simulink model "MPC_Observer_revised2"  (R2015a)
settings: Solver=ode5  StartTime=0.0  StopTime=Total_t_sim  FixedStep=dt  RelTol=1e-3
values from neighbouring files (symbols this model uses):
  A = F    [DMPC_AVC12.m]    (also in DMPC_AVC2.m; DMPC_AVC4.m; DMPC_AVC6.m)
  A_cons = [L_m;-L_m]    [DMPC_AVC12.m]    (also in DMPC_AVC2.m; DMPC_AVC4.m; DMPC_AVC6.m)
  A_nom = A    [DMPC_AVC12.m]    (also in DMPC_AVC2.m; DMPC_AVC4.m; DMPC_AVC6.m)
  B = G    [DMPC_AVC12.m]    (also in DMPC_AVC2.m; DMPC_AVC4.m; DMPC_AVC6.m)
  B_nom = B    [DMPC_AVC12.m]    (also in DMPC_AVC2.m; DMPC_AVC4.m; DMPC_AVC6.m)
  C = H    [DMPC_AVC12.m]    (also in DMPC_AVC2.m; DMPC_AVC4.m; DMPC_AVC6.m)
  C_nom = C    [DMPC_AVC12.m]    (also in DMPC_AVC2.m; DMPC_AVC4.m; DMPC_AVC6.m)
  coefs = coefs(1,2:end)    [DMPC_AVC12.m]    (also in DMPC_AVC2.m; DMPC_AVC4.m; DMPC_AVC6.m)
  dt = 5e-4    (= 0.0005)    [DMPC_AVC12.m]    (also in DMPC_AVC2.m = 0.001; DMPC_AVC4.m = 0.001; DMPC_AVC6.m = 0.001)
  H_nom = H    [DMPC_AVC12.m]    (also in DMPC_AVC2.m; DMPC_AVC4.m; DMPC_AVC6.m)
  Lf = Kalman_Gain(A,C,Qf,Rf,Pf,Nsim,nout)    [DMPC_AVC12.m]    (also in DMPC_AVC2.m; DMPC_AVC4.m; DMPC_AVC6.m)
  u_bound = [u_max;-u_min]    [DMPC_AVC12.m]    (also in DMPC_AVC2.m; DMPC_AVC4.m; DMPC_AVC6.m)
  V = gt_modal.C    [identification_SPM_IMP.m]    (also in identified_shaker.mat = [-0.780917041134 1.13362828061])
  W = gt_modal.A    [identification_SPM_IMP.m]    (also in identified_shaker.mat = [-1.30981674822  104.165252735; -104.165252735  -1.309816748)
undefined symbols (not defined in the file or in its folder): L_m, omega, psi
libraries: simulink_need_slupdate x2
settings Model: Creator=Ablah  LastModifiedBy=Ablah

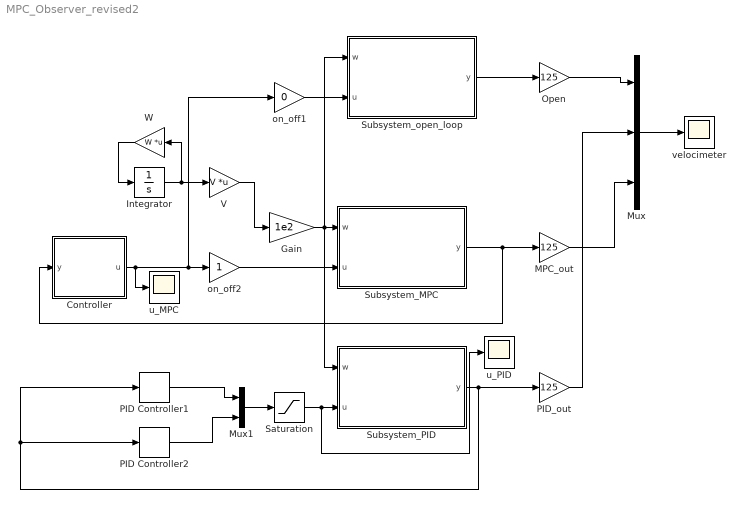
== system MPC_Observer_revised2 ==
  Controller : Subsystem
  Gain : Gain  Gain=1e2
  Integrator : Integrator  InitialCondition=0.01
  MPC_out : Gain  Gain=125
  Mux : Mux  Inputs=3
  Mux1 : Mux  Inputs=2
  Open : Gain  Gain=125
  PID Controller1 : simulink_need_slupdate/PID Controller  P=-3  I=-4  D=0
  PID Controller2 : simulink_need_slupdate/PID Controller  P=-3  I=-4  D=0
  PID_out : Gain  Gain=125
  Saturation : Saturate  UpperLimit=0.6  LowerLimit=-0.6
  Subsystem_MPC : Subsystem
  Subsystem_PID : Subsystem
  Subsystem_open_loop : Subsystem
  V : Gain  Gain=V  Multiplication=Matrix(K*u)
  W : Gain  Gain=W  Multiplication=Matrix(K*u)
  on_off1 : Gain  Gain=0
  on_off2 : Gain
  u_MPC : Scope
      settings: YMin=-2.25  YMax=2.25  SaveName=ScopeData5
  u_PID : Scope
      settings: YMin=-2.25  YMax=2.25  SaveName=ScopeData4
  velocimeter : Scope
      settings: ShowLegends=on  YMin=-10  YMax=10
  wires:
  Controller/1(u) -> u_MPC/1, on_off1/1, on_off2/1
  Gain/1 -> Subsystem_PID/1(w), Subsystem_open_loop/1(w), Subsystem_MPC/1(w)
  Subsystem_MPC/1(y) -> Controller/1(y), MPC_out/1
  on_off2/1 -> Subsystem_MPC/2(u)
  W/1 -> Integrator/1
  Integrator/1 -> V/1, W/1
  V/1 -> Gain/1
  on_off1/1 -> Subsystem_open_loop/2(u)
  Subsystem_open_loop/1(y) -> Open/1
  Mux/1 -> velocimeter/1
  Subsystem_PID/1(y) -> PID Controller2/1, PID Controller1/1, PID_out/1
  PID Controller1/1 -> Mux1/1
  Mux1/1 -> Saturation/1
  Saturation/1 -> u_PID/1, Subsystem_PID/2(u)
  PID Controller2/1 -> Mux1/2
  MPC_out/1 -> Mux/3
  Open/1 -> Mux/1
  PID_out/1 -> Mux/2

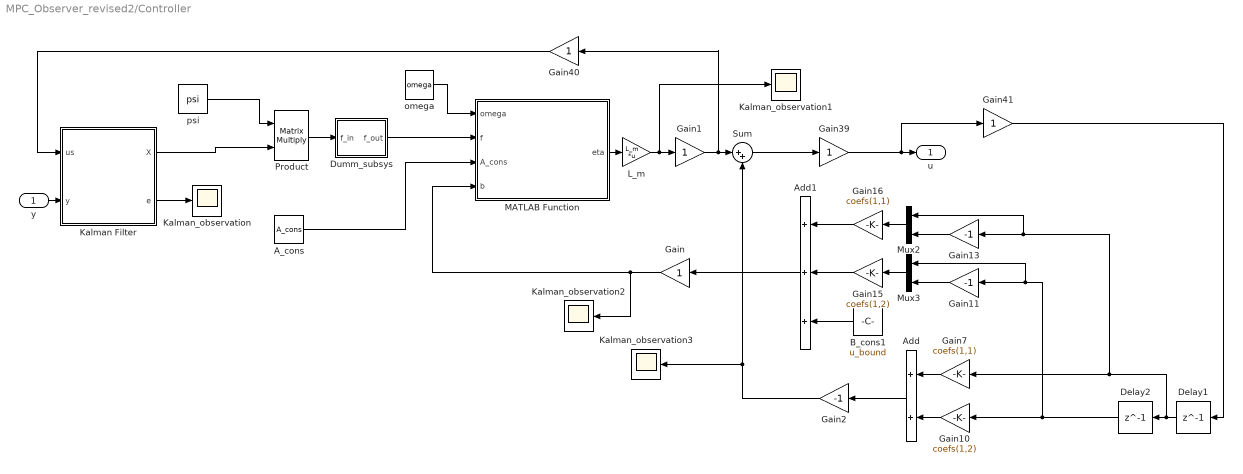
== system MPC_Observer_revised2/Controller ==
  y : Inport
  A_cons : Constant  Value=A_cons  SampleTime=dt
  Add : Sum
  Add1 : Sum  Inputs=+++
  B_cons1 : Constant  Value=u_bound
  Delay1 : Delay  DelayLength=1  InitialCondition=0  SampleTime=dt
  Delay2 : Delay  DelayLength=1  InitialCondition=0  SampleTime=dt
  Dumm_subsys : Subsystem
  Gain{,1,39..41} (5 alike) : Gain
  Gain10 : Gain  Gain=coefs(1,2)
  Gain11 : Gain  Gain=-1
  Gain13 : Gain  Gain=-1
  Gain15 : Gain  Gain=coefs(1,2)
  Gain16 : Gain  Gain=coefs(1,1)
  Gain2 : Gain  Gain=-1
  Gain7 : Gain  Gain=coefs(1,1)
  Kalman Filter : Subsystem  TreatAsAtomicUnit=on
      settings: MinAlgLoopOccurrences=on
  Kalman_observation{,1..3} (4 alike) : Scope
      Kalman_observation settings: YMin=-3.5e-11  YMax=3.5e-11
      Kalman_observation1 settings: YMin=-0.000155  YMax=-6.5e-05  SaveName=ScopeData2
      Kalman_observation2 settings: YMin=-0.000155  YMax=-6.5e-05  SaveName=ScopeData6
      Kalman_observation3 settings: YMin=-0.000155  YMax=-6.5e-05  SaveName=ScopeData7
  L_m : Gain  Gain=L_m  Multiplication=Matrix(K*u)
  MATLAB Function : MATLAB Function  TreatAsAtomicUnit=on
      settings: MinAlgLoopOccurrences=on
  Mux2 : Mux  Inputs=2
  Mux3 : Mux  Inputs=2
  Product : Product  Multiplication=Matrix(*)  RndMeth=Zero
  Sum : Sum  Inputs=|++
  omega : Constant  Value=omega  SampleTime=dt
  psi : Constant  Value=psi  SampleTime=dt
  u : Outport
  wires:
  MATLAB Function/1(eta) -> L_m/1
  L_m/1 -> Kalman_observation1/1, Gain1/1
  omega/1 -> MATLAB Function/1(omega)
  A_cons/1 -> MATLAB Function/3(A_cons)
  psi/1 -> Product/1
  y/1 -> Kalman Filter/2(y)
  Gain7/1 -> Add/1
  Gain13/1 -> Mux2/2
  Gain11/1 -> Mux3/2
  Mux2/1 -> Gain16/1
  Mux3/1 -> Gain15/1
  Gain16/1 -> Add1/1
  Gain15/1 -> Add1/2
  Add/1 -> Gain2/1
  Gain10/1 -> Add/2
  Product/1 -> Dumm_subsys/1(f_in)
  Dumm_subsys/1(f_out) -> MATLAB Function/2(f)
  Kalman Filter/1(X) -> Product/2
  Kalman Filter/2(e) -> Kalman_observation/1
  Gain1/1 -> Sum/1, Gain40/1
  Delay2/1 -> Mux3/1, Gain11/1, Gain10/1
  Delay1/1 -> Mux2/1, Gain13/1, Gain7/1, Delay2/1
  Sum/1 -> Gain39/1
  Gain2/1 -> Sum/2, Kalman_observation3/1
  Gain39/1 -> Gain41/1, u/1
  Gain40/1 -> Kalman Filter/1(us)
  Gain41/1 -> Delay1/1
  Add1/1 -> Gain/1
  Gain/1 -> Kalman_observation2/1, MATLAB Function/4(b)
  B_cons1/1 -> Add1/3

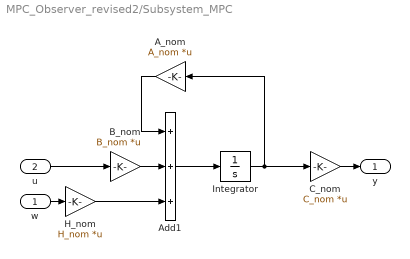
== system MPC_Observer_revised2/Subsystem_MPC ==
  w : Inport
  u : Inport  Port=2
  A_nom : Gain  Gain=A_nom  Multiplication=Matrix(K*u)
  Add1 : Sum  Inputs=+++
  B_nom : Gain  Gain=B_nom  Multiplication=Matrix(K*u)
  "C_nom " : Gain  Gain=C_nom  Multiplication=Matrix(K*u)
  H_nom : Gain  Gain=H_nom  Multiplication=Matrix(K*u)
  Integrator : Integrator
  y : Outport
  wires:
  "C_nom "/1 -> y/1
  Add1/1 -> Integrator/1
  A_nom/1 -> Add1/1
  H_nom/1 -> Add1/3
  Integrator/1 -> "C_nom "/1, A_nom/1
  B_nom/1 -> Add1/2
  u/1 -> B_nom/1
  w/1 -> H_nom/1

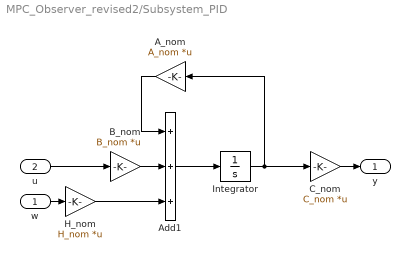
== system MPC_Observer_revised2/Subsystem_PID ==
  w : Inport
  u : Inport  Port=2
  A_nom : Gain  Gain=A_nom  Multiplication=Matrix(K*u)
  Add1 : Sum  Inputs=+++
  B_nom : Gain  Gain=B_nom  Multiplication=Matrix(K*u)
  "C_nom " : Gain  Gain=C_nom  Multiplication=Matrix(K*u)
  H_nom : Gain  Gain=H_nom  Multiplication=Matrix(K*u)
  Integrator : Integrator
  y : Outport
  wires:
  "C_nom "/1 -> y/1
  Add1/1 -> Integrator/1
  A_nom/1 -> Add1/1
  H_nom/1 -> Add1/3
  Integrator/1 -> "C_nom "/1, A_nom/1
  B_nom/1 -> Add1/2
  u/1 -> B_nom/1
  w/1 -> H_nom/1

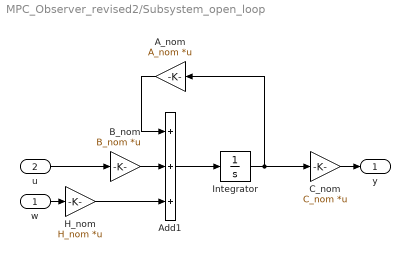
== system MPC_Observer_revised2/Subsystem_open_loop ==
  w : Inport
  u : Inport  Port=2
  A_nom : Gain  Gain=A_nom  Multiplication=Matrix(K*u)
  Add1 : Sum  Inputs=+++
  B_nom : Gain  Gain=B_nom  Multiplication=Matrix(K*u)
  "C_nom " : Gain  Gain=C_nom  Multiplication=Matrix(K*u)
  H_nom : Gain  Gain=H_nom  Multiplication=Matrix(K*u)
  Integrator : Integrator
  y : Outport
  wires:
  w/1 -> H_nom/1
  u/1 -> B_nom/1
  B_nom/1 -> Add1/2
  Integrator/1 -> A_nom/1, "C_nom "/1
  H_nom/1 -> Add1/3
  A_nom/1 -> Add1/1
  Add1/1 -> Integrator/1
  "C_nom "/1 -> y/1

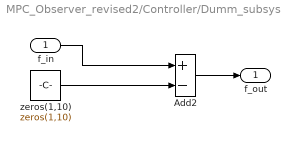
== system MPC_Observer_revised2/Controller/Dumm_subsys ==
  f_in : Inport
  Add2 : Sum  Inputs=+-
  zeros(1,10) : Constant  Value=zeros(1,10)  SampleTime=dt
  f_out : Outport
  wires:
  f_in/1 -> Add2/1
  Add2/1 -> f_out/1
  zeros(1,10)/1 -> Add2/2

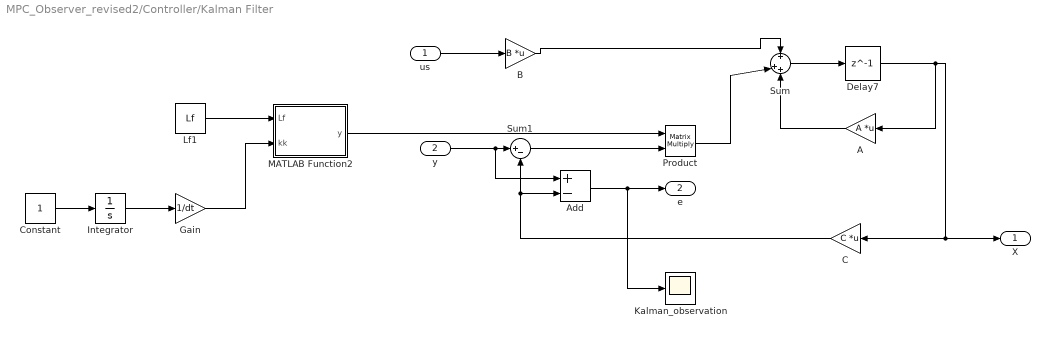
== system MPC_Observer_revised2/Controller/Kalman Filter ==
  us : Inport
  y : Inport  Port=2
  A : Gain  Gain=A  Multiplication=Matrix(K*u)
  Add : Sum  Inputs=+-
  B : Gain  Gain=B  Multiplication=Matrix(K*u)
  C : Gain  Gain=C  Multiplication=Matrix(K*u)
  Constant : Constant
  Delay7 : Delay  DelayLength=1  InitialCondition=0  SampleTime=dt
  Gain : Gain  Gain=1/dt
  Integrator : Integrator
  Kalman_observation : Scope
      settings: YMin=-8e-13  YMax=7e-13  SaveName=ScopeData3
  Lf1 : Constant  Value=Lf
  MATLAB Function2 : MATLAB Function  TreatAsAtomicUnit=on
      settings: MinAlgLoopOccurrences=on
  Product : Product  Multiplication=Matrix(*)  RndMeth=Zero
  Sum : Sum  Inputs=+|++
  Sum1 : Sum  Inputs=|+-
  X : Outport
  e : Outport  Port=2
  wires:
  Delay7/1 -> A/1, X/1, C/1
  A/1 -> Sum/3
  Sum/1 -> Delay7/1
  us/1 -> B/1
  B/1 -> Sum/1
  C/1 -> Add/2, Sum1/2
  y/1 -> Add/1, Sum1/1
  Sum1/1 -> Product/2
  Product/1 -> Sum/2
  Lf1/1 -> MATLAB Function2/1(Lf)
  MATLAB Function2/1(y) -> Product/1
  Constant/1 -> Integrator/1
  Integrator/1 -> Gain/1
  Gain/1 -> MATLAB Function2/2(kk)
  Add/1 -> Kalman_observation/1, e/1

== matlab function MPC_Observer_revised2/Controller/MATLAB Function ==
  data: omega input; eta output; f input; A_cons input; b input
function eta=QPomegaild(omega,f,A_cons,b)

[n1,m1]=size(A_cons);
% eta=-omega\f;
eta=-inv(omega)*f;
kk=0;
for i=1:n1
    if (A_cons(i,:)*eta>b(i)) 
        kk=kk+1;
    else
        kk=kk+0;
    end
end
if (kk==0)
    return
end
P=A_cons*(omega\A_cons');
d=(A_cons*(omega\f)+b);
[n,m]=size(d);
x_ini=zeros(n,m);
lambda=x_ini;
% al=10;
for km=1:38

%find tomegae elements in tomegae solution vector one by one
% km could be larger if tomegae Lagranger multiplier omegaas a slow
% convergence rate.
    lambda_p=lambda;
    for i=1:n
        w= P(i,:)*lambda-P(i,i)*lambda(i,1);
        w=w+d(i,1);
        la=-w/P(i,i);
        lambda(i,1)=max(0,la);
    end
    
    al=(lambda-lambda_p)'*(lambda-lambda_p);
    if (al<10e-30)
        break;
    end
 end
eta=-omega\f -omega\A_cons'*lambda;

== matlab function MPC_Observer_revised2/Controller/Kalman Filter/MATLAB Function2 ==
  data: y output; Lf input; kk input
function y = fcn(Lf,kk)
%#eml

kk1 = floor(kk)+1;

y = Lf(:,kk1);
% y = Lf;
